simulink model "pid_model_disc2"  (Simulink 8.1)
settings: Solver=ode4  StartTime=0.0  StopTime=5000.0  FixedStep=0.2  RelTol=1e-3
libraries: simulink x1
settings Model: Creator=Avega  LastModifiedBy=Avega
settings DataIOCC: SignalLoggingSaveFormat=Dataset
settings OptimizationCC: ExpressionDepthLimit=128

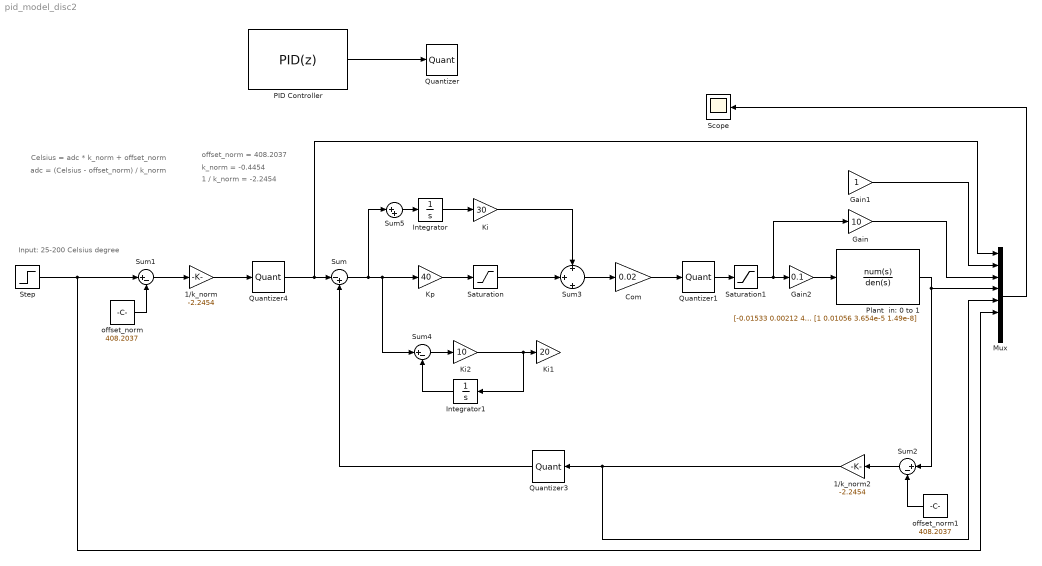
== system pid_model_disc2 ==
  note: 1 / k_norm = -2.2454
  note: k_norm = -0.4454
  note: offset_norm = 408.2037
  note: adc = (Celsius - offset_norm) / k_norm
  note: Celsius = adc * k_norm + offset_norm
  note: Input: 25-200 Celsius degree
  1/k_norm : Gain  Gain=-2.2454
  1/k_norm2 : Gain  Gain=-2.2454
  Com : Gain  Gain=0.02
  Gain : Gain  Gain=10
  Gain1 : Gain
  Gain2 : Gain  Gain=0.1
  Integrator : Integrator  LimitOutput=on  UpperSaturationLimit=10  LowerSaturationLimit=-10
  Integrator1 : Integrator  LimitOutput=on  UpperSaturationLimit=100  LowerSaturationLimit=-100
  Ki : Gain  Gain=30
  Ki1 : Gain  Gain=20
  Ki2 : Gain  Gain=10
  Kp : Gain  Gain=40
  Mux : Mux  Inputs=8
  PID Controller : simulink/Continuous/PID Controller  Controller=PID  TimeDomain=Discrete-time  SampleTime=0.2  IntegratorMethod=Forward Euler  FilterMethod=Forward Euler  Form=Parallel  P=0.167429214907763  I=0.000126480289546085  D=16.0468346075827  N=5.17110660582003  InitialConditionSource=internal  InitialConditionForIntegrator=0  InitialConditionForFilter=0  ExternalReset=none  ZeroCross=off  LimitOutput=on  UpperSaturationLimit=1  LowerSaturationLimit=0  LinearizeAsGain=off  AntiWindupMode=clamping  Kb=1  TrackingMode=off  Kt=1  PParamMin=[]  PParamMax=[]  IParamMin=[]  IParamMax=[]  DParamMin=[]  DParamMax=[]  NParamMin=[]  NParamMax=[]  KbParamMin=[]  KbParamMax=[]  KtParamMin=[]  KtParamMax=[]  POutMin=[]  POutMax=[]  IOutMin=[]  IOutMax=[]  DOutMin=[]  DOutMax=[]  NOutMin=[]  NOutMax=[]  KbOutMin=[]  KbOutMax=[]  KtOutMin=[]  KtOutMax=[]  IntegratorOutMin=[]  IntegratorOutMax=[]  FilterOutMin=[]  FilterOutMax=[]  SumOutMin=[]  SumOutMax=[]  SumI1OutMin=[]  SumI1OutMax=[]  SumI2OutMin=[]  SumI2OutMax=[]  SumI3OutMin=[]  SumI3OutMax=[]  SumDOutMin=[]  SumDOutMax=[]  SaturationOutMin=[]  SaturationOutMax=[]  IntegratorContinuousStateAttributes=''  IntegratorStateMustResolveToSignalObject=off  IntegratorRTWStateStorageClass=Auto  FilterContinuousStateAttributes=''  FilterStateMustResolveToSignalObject=off  FilterRTWStateStorageClass=Auto
  Plant  in: 0 to 1 : TransferFcn  Numerator=[-0.01533 0.00212 4.827e-6]  Denominator=[1 0.01056 3.654e-5 1.49e-8]
  Quantizer : Quantizer  QuantizationInterval=0.1  LinearizeAsGain=off
  Quantizer1 : Quantizer  QuantizationInterval=1  LinearizeAsGain=off
  Quantizer3 : Quantizer  QuantizationInterval=1  LinearizeAsGain=off
  Quantizer4 : Quantizer  QuantizationInterval=1  LinearizeAsGain=off
  Saturation : Saturate  UpperLimit=8191  LowerLimit=-8192
  Saturation1 : Saturate  UpperLimit=10  LowerLimit=0
  Scope : Scope
      settings: TimeRange=3000  YMin=-20  YMax=180
  Step : Step  Time=2500  Before=150  After=100
  Sum : Sum  Inputs=|-+
  Sum1 : Sum  Inputs=|+-
  Sum2 : Sum  Inputs=|+-
  Sum3 : Sum  Inputs=+|+|+
  Sum4 : Sum  Inputs=|+-
  Sum5 : Sum  Inputs=|++
  offset_norm : Constant  Value=408.2037
  offset_norm1 : Constant  Value=408.2037
  wires:
  offset_norm/1 -> Sum1/2
  Step/1 -> Mux/6, Sum1/1
  Sum1/1 -> 1/k_norm/1
  offset_norm1/1 -> Sum2/2
  Sum2/1 -> 1/k_norm2/1
  Plant  in: 0 to 1/1 -> Sum2/1, Mux/4
  1/k_norm/1 -> Quantizer4/1
  1/k_norm2/1 -> Mux/5, Quantizer3/1
  Gain/1 -> Mux/3
  Gain1/1 -> Mux/2
  Kp/1 -> Saturation/1
  PID Controller/1 -> Quantizer/1
  Gain2/1 -> Plant  in: 0 to 1/1
  Saturation/1 -> Sum3/2
  Integrator/1 -> Ki/1
  Sum3/1 -> Com/1
  Saturation1/1 -> Gain/1, Gain2/1
  Quantizer4/1 -> Mux/1, Sum/1
  Com/1 -> Quantizer1/1
  Mux/1 -> Scope/1
  Ki/1 -> Sum3/1
  Quantizer1/1 -> Saturation1/1
  Quantizer3/1 -> Sum/2
  Sum5/1 -> Integrator/1
  Sum/1 -> Sum5/1, Sum4/1, Kp/1
  Sum4/1 -> Ki2/1
  Integrator1/1 -> Sum4/2
  Ki2/1 -> Integrator1/1, Ki1/1
